simulink model "simulink_Rositani"  (R2023b)
settings: Solver=VariableStepAuto  StartTime=0.0  StopTime=10  RelTol=1e-3
values from neighbouring files (symbols this model uses):
  A_lin = [   0                       1       0       0 ... (first row only)    [main_Rositani.m]
  B_lin = [   0   0   0   1/Jm]'    [main_Rositani.m]
  Beta = sym2poly(X)    [main_Rositani.m]
  Beta_integrator = sym2poly(X_integrator)    [main_Rositani.m]
  Bl = 0    [main_Rositani.m]
  Bm = 0.015    [main_Rositani.m]
  C_lin = [   1   0   0   0]    [main_Rositani.m]
  Cfl = [1 0 0 0]    [main_Rositani.m]
  Cfl_ext = [Cfl 0]    [main_Rositani.m]
  D_lin = 0    [main_Rositani.m]
  Dfl = 0    [main_Rositani.m]
  g = 9.8    [main_Rositani.m]
  Jl = 4e-4    (= 0.0004)    [main_Rositani.m]
  Jm = Jl    (= 0.0004)    [main_Rositani.m]
  k = 0.8    [main_Rositani.m]
  Kobs = place(A_lin',C_lin',[-200,-250,-300,-350])'    [main_Rositani.m]
  Kobsfl = place(M',Cfl',[-200,-250,-300,-350])'    [main_Rositani.m]
  Kobsfl_VSCext = place(M_VSCext',Cfl_ext',[-200,-250,-300,-350,-400])'    [main_Rositani.m]
  kppext = place(Aext,Bext,[-20 -25 -30 -35 -40])    [main_Rositani.m]
  kppext_fl = place(Mext,Next,[-20 -25 -30 -35 -40])    [main_Rositani.m]
  l = 0.3    [main_Rositani.m]
  M = [0 1 0 0;0 0 1 0; 0 0 0 1; 0 0 0 0]    [main_Rositani.m]
  m = 0.3    [main_Rositani.m]
  M_VSCext = [M N;zeros(1,5)]    [main_Rositani.m]
  N = [0;0;0;1]    [main_Rositani.m]
  q = 10    [main_Rositani.m]
  r = 100    [main_Rositani.m]
  step_amp = pi/4+pi/8    (= 1.1780972451)    [main_Rositani.m]
  u_bar = m*g*l*cos(pi/4)    [main_Rositani.m]
  x0 = [x1_bar,0,x3_bar,0]'    [main_Rositani.m]
  x1_bar = pi/4    (= 0.785398163397)    [main_Rositani.m]
  x3_bar = m*g*l/k*cos(pi/4)+pi/4    [main_Rositani.m]
settings Model: Creator=gtost  LastModifiedBy=marco
settings SolverCC: ZeroCrossAlgorithm=Adaptive
settings OptimizationCC: ReuseModelBlockBuffer=off
settings DebuggingCC: MaskedZcDiagnostic=none  IgnoredZcDiagnostic=none

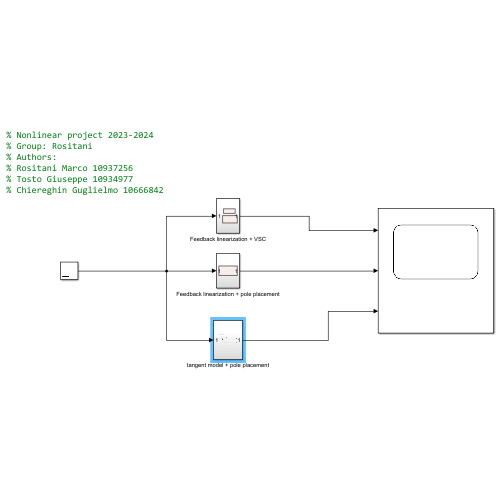
[thumbnail: Simulink's stored preview of the top-level diagram]
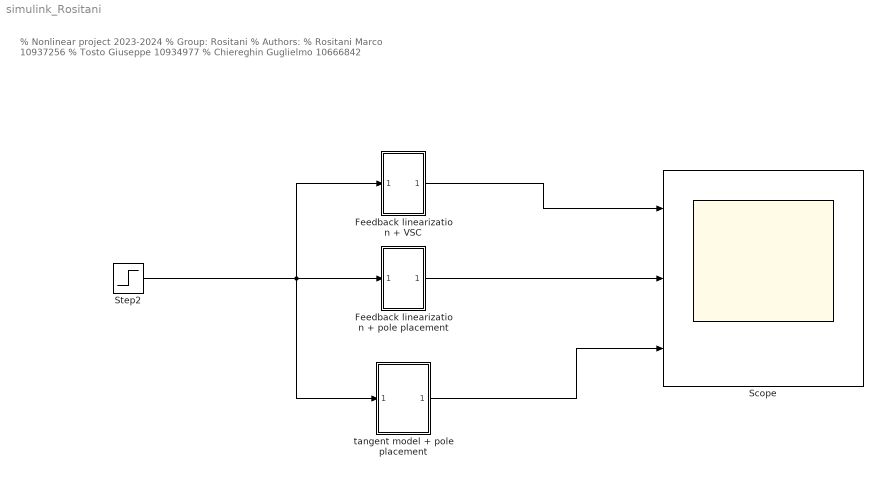
== system simulink_Rositani ==
  note: % Nonlinear project 2023-2024
      | % Group: Rositani
      | % Authors:
      | % Rositani Marco 10937256
      | % Tosto Giuseppe 10934977
      | % Chiereghin Guglielmo 10666842
  Feedback linearization + VSC : Subsystem
  Feedback linearization + pole placement : Subsystem
  Scope : Scope  NumInputPorts=3
  Step2 : Step  After=step_amp  SampleTime=0
  tangent model + pole placement : Subsystem
  wires:
  Feedback linearization + pole placement/1(Out1) -> Scope/2
  Feedback linearization + VSC/1(Out2) -> Scope/1
  tangent model + pole placement/1(Out1) -> Scope/3
  Step2/1 -> Feedback linearization + pole placement/1(Input), tangent model + pole placement/1(Input), Feedback linearization + VSC/1(Input)

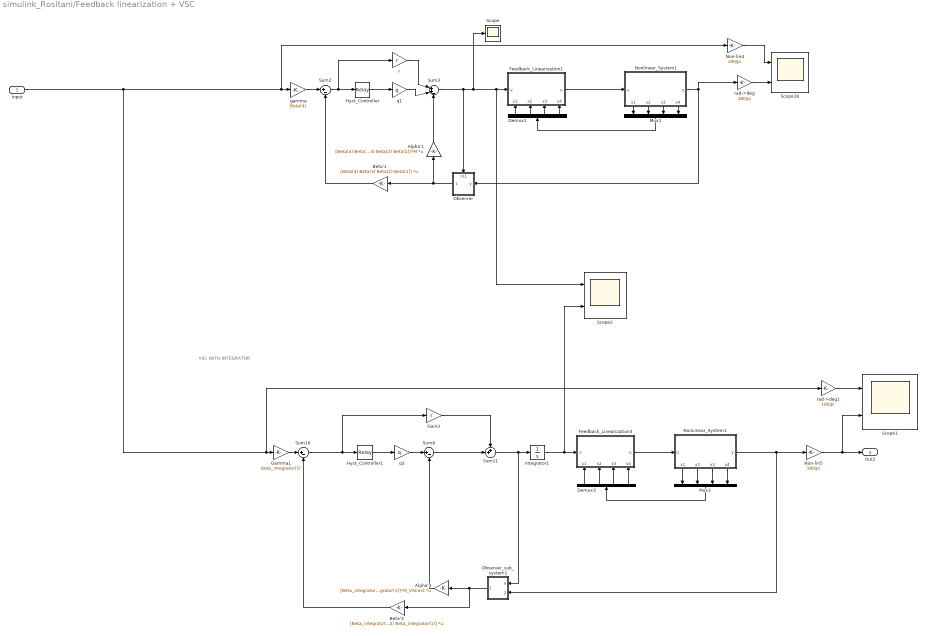
== system simulink_Rositani/Feedback linearization + VSC ==
  note: VSC WITH INTEGRATOR
  Input : Inport
  Alpha'1 : Gain  Gain=[Beta(4) Beta(3) Beta(2) Beta(1)]*M  Multiplication=Matrix(K*u)
  Alpha'3 : Gain  Gain=[Beta_integrator(5) Beta_integrator(4) Beta_integrator(3) Beta_integrator(2) Beta_integrator(1)]*M_VSCext  Multiplication=Matrix(K*u)
  Beta'1 : Gain  Gain=[Beta(4) Beta(3) Beta(2) Beta(1)]  Multiplication=Matrix(K*u)
  Beta'3 : Gain  Gain=[Beta_integrator(5) Beta_integrator(4) Beta_integrator(3) Beta_integrator(2) Beta_integrator(1)]  Multiplication=Matrix(K*u)
  Demux1 : Demux
  Demux3 : Demux
  Feedback_Linearization1 : Subsystem
      settings: PortSchema="{\"entries\":[{\"content\":{\"sides\":[{\"content\":{\"connectorIds\":[\"In1\",\"In2\",\"In3\",\"In4\"]},\"type\":\"ConnectorPlacement.EquallySpacedRectSide\",\"uuid\":\"adbcf6e9-d4ea-42de-99ff-13edcb3b1819\"},{\"content\":{\"connectorIds\":[],\"side\":\"RIGHT\"},\"type\":\"ConnectorPlacement.EquallySpacedRectSide\",\"uuid\":\"b525c529-ac30-4eee-aa98-8a0e478b5fb8\"},{\"content\":{\"connectorIds\":[\"In5\"],\"side\":\"TOP\"},\"type\":\"ConnectorPlacement.EquallySpacedRectSide\",\"uuid\":\"f99f0ac5-025d-4a5c-b3b2-d4280c578d78\"},{\"content\":{\"connectorIds\":[\"Out1\"],\"side\":\"BOTTOM\"},\"type\":\"ConnectorPlacement.EquallySpacedRectSide\",\"uuid\":\"0062a15c-7fea-4434-a819-637327a8425c\"}]},\"type\":\"ConnectorPlacement.EquallySpacedConnector\",\"uuid\":\"4fadabde-502f-417b-a41d-67ea1bbf08a5\"}],\"packageUris\":[\"http://schema.mathworks.com/mf0/Connector/R2020b\"],\"version\":\"1.0\"}"
  Feedback_Linearization3 : Subsystem
      settings: PortSchema="{\"entries\":[{\"content\":{\"sides\":[{\"content\":{\"connectorIds\":[\"In1\",\"In2\",\"In3\",\"In4\"]},\"type\":\"ConnectorPlacement.EquallySpacedRectSide\",\"uuid\":\"adbcf6e9-d4ea-42de-99ff-13edcb3b1819\"},{\"content\":{\"connectorIds\":[],\"side\":\"RIGHT\"},\"type\":\"ConnectorPlacement.EquallySpacedRectSide\",\"uuid\":\"b525c529-ac30-4eee-aa98-8a0e478b5fb8\"},{\"content\":{\"connectorIds\":[\"In5\"],\"side\":\"TOP\"},\"type\":\"ConnectorPlacement.EquallySpacedRectSide\",\"uuid\":\"f99f0ac5-025d-4a5c-b3b2-d4280c578d78\"},{\"content\":{\"connectorIds\":[\"Out1\"],\"side\":\"BOTTOM\"},\"type\":\"ConnectorPlacement.EquallySpacedRectSide\",\"uuid\":\"0062a15c-7fea-4434-a819-637327a8425c\"}]},\"type\":\"ConnectorPlacement.EquallySpacedConnector\",\"uuid\":\"4fadabde-502f-417b-a41d-67ea1bbf08a5\"}],\"packageUris\":[\"http://schema.mathworks.com/mf0/Connector/R2020b\"],\"version\":\"1.0\"}"
  Gain3 : Gain  Gain=r
  Gamma1 : Gain  Gain=Beta_integrator(5)
  Hyst_Controller : Relay  OnSwitchValue=0.2  OffSwitchValue=-0.2  OffOutputValue=-1
  Hyst_Controller1 : Relay  OnSwitchValue=0.2  OffSwitchValue=-0.2  OffOutputValue=-1
  Integrator1 : Integrator
  Mux1 : Mux
  Mux3 : Mux
  Non-lin4 : Gain  Gain=180/pi
  Non-lin5 : Gain  Gain=180/pi
  NonLInear_System1 : Subsystem
      settings: PortSchema="{\"entries\":[{\"content\":{\"sides\":[{\"content\":{\"connectorIds\":[]},\"type\":\"ConnectorPlacement.EquallySpacedRectSide\",\"uuid\":\"fc0e07bd-457d-4f73-a9de-b189f04b7406\"},{\"content\":{\"connectorIds\":[\"Out1\",\"Out2\",\"Out3\",\"Out4\"],\"side\":\"RIGHT\"},\"type\":\"ConnectorPlacement.EquallySpacedRectSide\",\"uuid\":\"a5405dd1-72e2-47e5-bf61-3afb592fd614\"},{\"content\":{\"connectorIds\":[\"In1\"],\"side\":\"TOP\"},\"type\":\"ConnectorPlacement.EquallySpacedRectSide\",\"uuid\":\"aa9f9cfa-860e-40f5-842c-a49042685ea7\"},{\"content\":{\"connectorIds\":[\"Out5\"],\"side\":\"BOTTOM\"},\"type\":\"ConnectorPlacement.EquallySpacedRectSide\",\"uuid\":\"187ae16a-996b-4444-8d39-d1043468c76c\"}]},\"type\":\"ConnectorPlacement.EquallySpacedConnector\",\"uuid\":\"6dd1d8f9-1d62-4e9a-bec2-4b959d6b58c0\"}],\"packageUris\":[\"http://schema.mathworks.com/mf0/Connector/R2020b\"],\"version\":\"1.0\"}"
  Nonlinear_System1 : Subsystem
      settings: PortSchema="{\"entries\":[{\"content\":{\"sides\":[{\"content\":{\"connectorIds\":[]},\"type\":\"ConnectorPlacement.EquallySpacedRectSide\",\"uuid\":\"fc0e07bd-457d-4f73-a9de-b189f04b7406\"},{\"content\":{\"connectorIds\":[\"Out1\",\"Out2\",\"Out3\",\"Out4\"],\"side\":\"RIGHT\"},\"type\":\"ConnectorPlacement.EquallySpacedRectSide\",\"uuid\":\"a5405dd1-72e2-47e5-bf61-3afb592fd614\"},{\"content\":{\"connectorIds\":[\"In1\"],\"side\":\"TOP\"},\"type\":\"ConnectorPlacement.EquallySpacedRectSide\",\"uuid\":\"aa9f9cfa-860e-40f5-842c-a49042685ea7\"},{\"content\":{\"connectorIds\":[\"Out5\"],\"side\":\"BOTTOM\"},\"type\":\"ConnectorPlacement.EquallySpacedRectSide\",\"uuid\":\"187ae16a-996b-4444-8d39-d1043468c76c\"}]},\"type\":\"ConnectorPlacement.EquallySpacedConnector\",\"uuid\":\"6dd1d8f9-1d62-4e9a-bec2-4b959d6b58c0\"}],\"packageUris\":[\"http://schema.mathworks.com/mf0/Connector/R2020b\"],\"version\":\"1.0\"}"
  Observer : Subsystem
      settings: PortSchema="{\"entries\":[{\"content\":{\"sides\":[{\"content\":{\"connectorIds\":[\"In1\"]},\"type\":\"ConnectorPlacement.EquallySpacedRectSide\",\"uuid\":\"2b2df3d8-1279-46b4-93b2-b5e918df1143\"},{\"content\":{\"connectorIds\":[\"Out1\"],\"side\":\"RIGHT\"},\"type\":\"ConnectorPlacement.EquallySpacedRectSide\",\"uuid\":\"29834a7d-bd18-478f-8842-72b452eb8ac1\"},{\"content\":{\"connectorIds\":[\"In2\"],\"side\":\"TOP\"},\"type\":\"ConnectorPlacement.EquallySpacedRectSide\",\"uuid\":\"8e28432d-3188-4e3a-b594-25bb706f296d\"}]},\"type\":\"ConnectorPlacement.EquallySpacedConnector\",\"uuid\":\"3baf92a3-067b-448e-904e-78e17b82779c\"}],\"packageUris\":[\"http://schema.mathworks.com/mf0/Connector/R2020b\"],\"version\":\"1.0\"}"
  Observer_sub_system1 : Subsystem
  Scope : Scope
  Scope1 : Scope  NumInputPorts=2
  Scope18 : Scope  NumInputPorts=2
  Scope2 : Scope  NumInputPorts=2
  Sum10 : Sum  Inputs=|+-
  Sum11 : Sum  Inputs=++|
  Sum2 : Sum  Inputs=|+-
  Sum3 : Sum  Inputs=|++-
  Sum8 : Sum  Inputs=|+-
  gamma : Gain  Gain=Beta(4)
  q1 : Gain  Gain=q
  q3 : Gain  Gain=q
  r : Gain  Gain=r
  rad->deg : Gain  Gain=180/pi
  rad->deg1 : Gain  Gain=180/pi
  Out2 : Outport
  wires:
  Non-lin4/1 -> Scope18/1
  Beta'1/1 -> Sum2/2
  rad->deg/1 -> Scope18/2
  Hyst_Controller/1 -> q1/1
  gamma/1 -> Sum2/1
  Nonlinear_System1/5(y) -> rad->deg/1, Observer/1(y)
  Nonlinear_System1/2(x2) -> Mux1/2
  Input/1 -> Non-lin4/1, gamma/1, rad->deg1/1, Gamma1/1
  Sum2/1 -> r/1, Hyst_Controller/1
  q1/1 -> Sum3/2
  Sum3/1 -> Observer/2(In1), Scope2/1, Feedback_Linearization1/5(v), Scope/1
  Mux1/1 -> Demux1/1
  Observer/1(Out1) -> Beta'1/1, Alpha'1/1
  Alpha'1/1 -> Sum3/3
  Nonlinear_System1/3(x3) -> Mux1/3
  Demux1/1 -> Feedback_Linearization1/1(x1)
  Nonlinear_System1/1(x1) -> Mux1/1
  r/1 -> Sum3/1
  Demux1/3 -> Feedback_Linearization1/3(x3)
  Demux1/2 -> Feedback_Linearization1/2(x2)
  Demux1/4 -> Feedback_Linearization1/4(x4)
  Nonlinear_System1/4(x4) -> Mux1/4
  Feedback_Linearization1/1(u) -> Nonlinear_System1/1(u)
  Alpha'3/1 -> Sum8/2
  Feedback_Linearization3/1(u) -> NonLInear_System1/1(u)
  Sum11/1 -> Integrator1/1, Observer_sub_system1/1(u)
  q3/1 -> Sum8/1
  Hyst_Controller1/1 -> q3/1
  Gamma1/1 -> Sum10/1
  Non-lin5/1 -> Scope1/2, Out2/1
  NonLInear_System1/3(x3) -> Mux3/3
  Gain3/1 -> Sum11/1
  NonLInear_System1/5(y) -> Observer_sub_system1/2(Input), Non-lin5/1
  Observer_sub_system1/1(Out1) -> Alpha'3/1, Beta'3/1
  Sum10/1 -> Hyst_Controller1/1, Gain3/1
  Demux3/2 -> Feedback_Linearization3/2(x2)
  NonLInear_System1/2(x2) -> Mux3/2
  NonLInear_System1/4(x4) -> Mux3/4
  Demux3/3 -> Feedback_Linearization3/3(x3)
  Mux3/1 -> Demux3/1
  Beta'3/1 -> Sum10/2
  Demux3/1 -> Feedback_Linearization3/1(x1)
  Sum8/1 -> Sum11/2
  NonLInear_System1/1(x1) -> Mux3/1
  Demux3/4 -> Feedback_Linearization3/4(x4)
  rad->deg1/1 -> Scope1/1
  Integrator1/1 -> Scope2/2, Feedback_Linearization3/5(v)

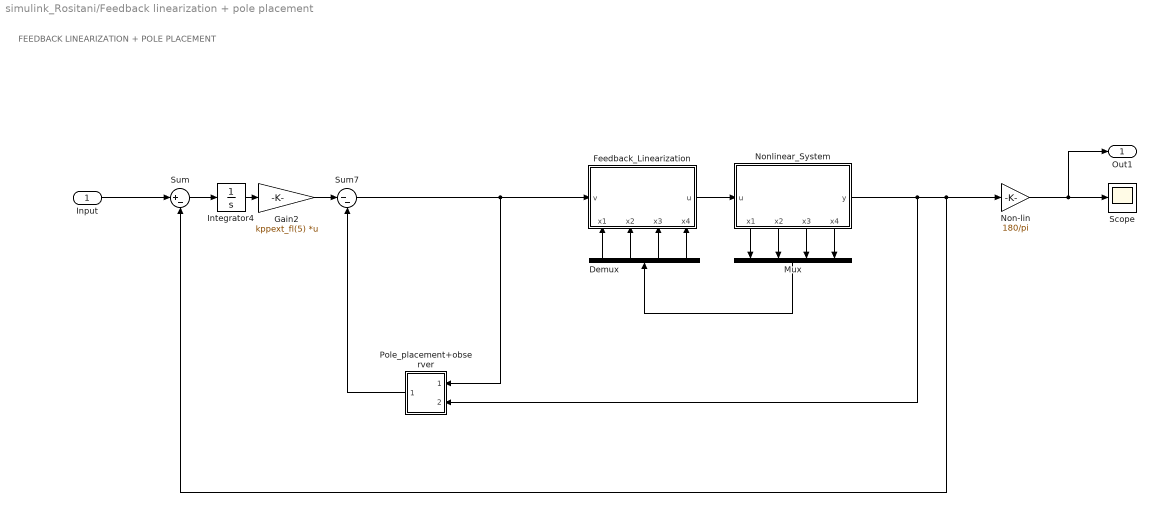
== system simulink_Rositani/Feedback linearization + pole placement ==
  note: FEEDBACK LINEARIZATION + POLE PLACEMENT
  Input : Inport
  Demux : Demux
  Feedback_Linearization : Subsystem
      settings: PortSchema="{\"entries\":[{\"content\":{\"sides\":[{\"content\":{\"connectorIds\":[\"In1\",\"In2\",\"In3\",\"In4\"]},\"type\":\"ConnectorPlacement.EquallySpacedRectSide\",\"uuid\":\"adbcf6e9-d4ea-42de-99ff-13edcb3b1819\"},{\"content\":{\"side\":\"RIGHT\"},\"type\":\"ConnectorPlacement.EquallySpacedRectSide\",\"uuid\":\"b525c529-ac30-4eee-aa98-8a0e478b5fb8\"},{\"content\":{\"connectorIds\":[\"In5\"],\"side\":\"TOP\"},\"type\":\"ConnectorPlacement.EquallySpacedRectSide\",\"uuid\":\"f99f0ac5-025d-4a5c-b3b2-d4280c578d78\"},{\"content\":{\"connectorIds\":[\"Out1\"],\"side\":\"BOTTOM\"},\"type\":\"ConnectorPlacement.EquallySpacedRectSide\",\"uuid\":\"0062a15c-7fea-4434-a819-637327a8425c\"}]},\"type\":\"ConnectorPlacement.EquallySpacedConnector\",\"uuid\":\"4fadabde-502f-417b-a41d-67ea1bbf08a5\"}],\"packageUris\":[\"http://schema.mathworks.com/mf0/Connector/R2020b\"],\"version\":\"1.0\"}"
  Gain2 : Gain  Gain=kppext_fl(5)  Multiplication=Matrix(K*u) (u vector)
  Integrator4 : Integrator
  Mux : Mux
  Non-lin : Gain  Gain=180/pi
  Nonlinear_System : Subsystem
      settings: PortSchema="{\"entries\":[{\"content\":{\"sides\":[{\"content\":{\"connectorIds\":[]},\"type\":\"ConnectorPlacement.EquallySpacedRectSide\",\"uuid\":\"fc0e07bd-457d-4f73-a9de-b189f04b7406\"},{\"content\":{\"connectorIds\":[\"Out1\",\"Out2\",\"Out3\",\"Out4\"],\"side\":\"RIGHT\"},\"type\":\"ConnectorPlacement.EquallySpacedRectSide\",\"uuid\":\"a5405dd1-72e2-47e5-bf61-3afb592fd614\"},{\"content\":{\"connectorIds\":[\"In1\"],\"side\":\"TOP\"},\"type\":\"ConnectorPlacement.EquallySpacedRectSide\",\"uuid\":\"aa9f9cfa-860e-40f5-842c-a49042685ea7\"},{\"content\":{\"connectorIds\":[\"Out5\"],\"side\":\"BOTTOM\"},\"type\":\"ConnectorPlacement.EquallySpacedRectSide\",\"uuid\":\"187ae16a-996b-4444-8d39-d1043468c76c\"}]},\"type\":\"ConnectorPlacement.EquallySpacedConnector\",\"uuid\":\"6dd1d8f9-1d62-4e9a-bec2-4b959d6b58c0\"}],\"packageUris\":[\"http://schema.mathworks.com/mf0/Connector/R2020b\"],\"version\":\"1.0\"}"
  Pole_placement+observer : Subsystem
  Scope : Scope
  Sum : Sum  Inputs=|+-
  Sum7 : Sum  Inputs=|--
  Out1 : Outport
  wires:
  Nonlinear_System/2(x2) -> Mux/2
  Demux/1 -> Feedback_Linearization/1(x1)
  Demux/4 -> Feedback_Linearization/4(x4)
  Pole_placement+observer/1(Out1) -> Sum7/2
  Nonlinear_System/1(x1) -> Mux/1
  Gain2/1 -> Sum7/1
  Sum7/1 -> Pole_placement+observer/1(In1), Feedback_Linearization/5(v)
  Nonlinear_System/4(x4) -> Mux/4
  Nonlinear_System/3(x3) -> Mux/3
  Demux/3 -> Feedback_Linearization/3(x3)
  Demux/2 -> Feedback_Linearization/2(x2)
  Sum/1 -> Integrator4/1
  Nonlinear_System/5(y) -> Pole_placement+observer/2(Input), Sum/2, Non-lin/1
  Integrator4/1 -> Gain2/1
  Feedback_Linearization/1(u) -> Nonlinear_System/1(u)
  Non-lin/1 -> Scope/1, Out1/1
  Input/1 -> Sum/1
  Mux/1 -> Demux/1

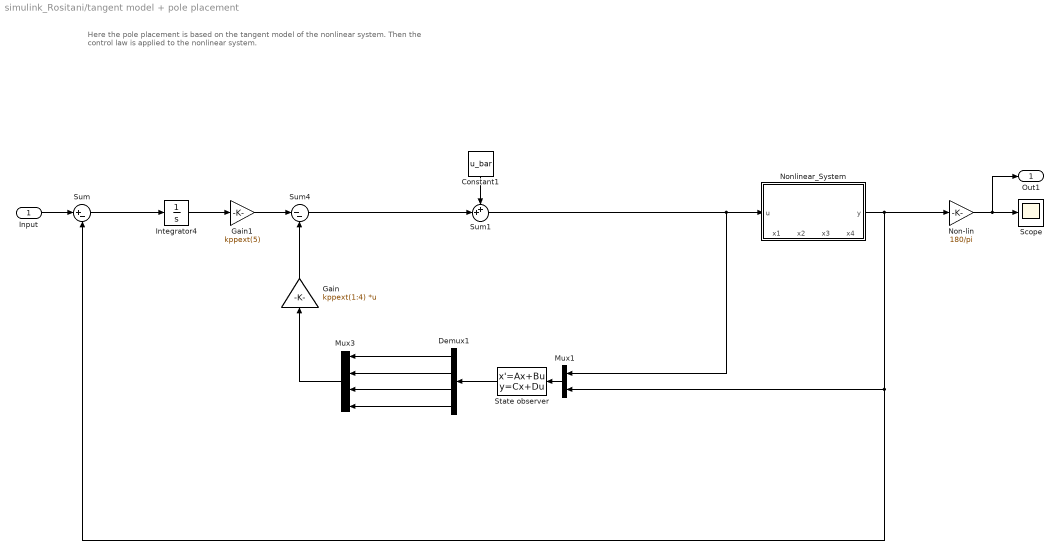
== system simulink_Rositani/tangent model + pole placement ==
  note: Here the pole placement is based on the tangent model of the nonlinear system. Then the control law is applied to the nonlinear system.
  Input : Inport
  Constant1 : Constant  Value=u_bar
  Demux1 : Demux
  Gain : Gain  Gain=kppext(1:4)  Multiplication=Matrix(K*u) (u vector)
  Gain1 : Gain  Gain=kppext(5)
  Integrator4 : Integrator
  Mux1 : Mux  Inputs=2
  Mux3 : Mux
  Non-lin : Gain  Gain=180/pi
  Nonlinear_System : Subsystem
      settings: PortSchema="{\"entries\":[{\"content\":{\"sides\":[{\"content\":{\"connectorIds\":[]},\"type\":\"ConnectorPlacement.EquallySpacedRectSide\",\"uuid\":\"fc0e07bd-457d-4f73-a9de-b189f04b7406\"},{\"content\":{\"connectorIds\":[\"Out1\",\"Out2\",\"Out3\",\"Out4\"],\"side\":\"RIGHT\"},\"type\":\"ConnectorPlacement.EquallySpacedRectSide\",\"uuid\":\"a5405dd1-72e2-47e5-bf61-3afb592fd614\"},{\"content\":{\"connectorIds\":[\"In1\"],\"side\":\"TOP\"},\"type\":\"ConnectorPlacement.EquallySpacedRectSide\",\"uuid\":\"aa9f9cfa-860e-40f5-842c-a49042685ea7\"},{\"content\":{\"connectorIds\":[\"Out5\"],\"side\":\"BOTTOM\"},\"type\":\"ConnectorPlacement.EquallySpacedRectSide\",\"uuid\":\"187ae16a-996b-4444-8d39-d1043468c76c\"}]},\"type\":\"ConnectorPlacement.EquallySpacedConnector\",\"uuid\":\"6dd1d8f9-1d62-4e9a-bec2-4b959d6b58c0\"}],\"packageUris\":[\"http://schema.mathworks.com/mf0/Connector/R2020b\"],\"version\":\"1.0\"}"
  Scope : Scope
  State observer : StateSpace  A=A_lin-Kobs*C_lin  B=[B_lin-Kobs*D_lin Kobs]  C=eye(4)  D=[0 0;0 0;0 0;0 0]  InitialCondition=0  ParameterTunability=Unconstrained
  Sum : Sum  Inputs=|+-
  Sum1 : Sum  Inputs=++|
  Sum4 : Sum  Inputs=|--
  Out1 : Outport
  wires:
  Sum4/1 -> Sum1/2
  Constant1/1 -> Sum1/1
  Sum1/1 -> Mux1/1, Nonlinear_System/1(u)
  State observer/1 -> Demux1/1
  Demux1/2 -> Mux3/2
  Demux1/4 -> Mux3/4
  Gain/1 -> Sum4/2
  Nonlinear_System/5(y) -> Non-lin/1, Sum/2, Mux1/2
  Sum/1 -> Integrator4/1
  Integrator4/1 -> Gain1/1
  Gain1/1 -> Sum4/1
  Mux1/1 -> State observer/1
  Demux1/1 -> Mux3/1
  Demux1/3 -> Mux3/3
  Non-lin/1 -> Out1/1, Scope/1
  Mux3/1 -> Gain/1
  Input/1 -> Sum/1

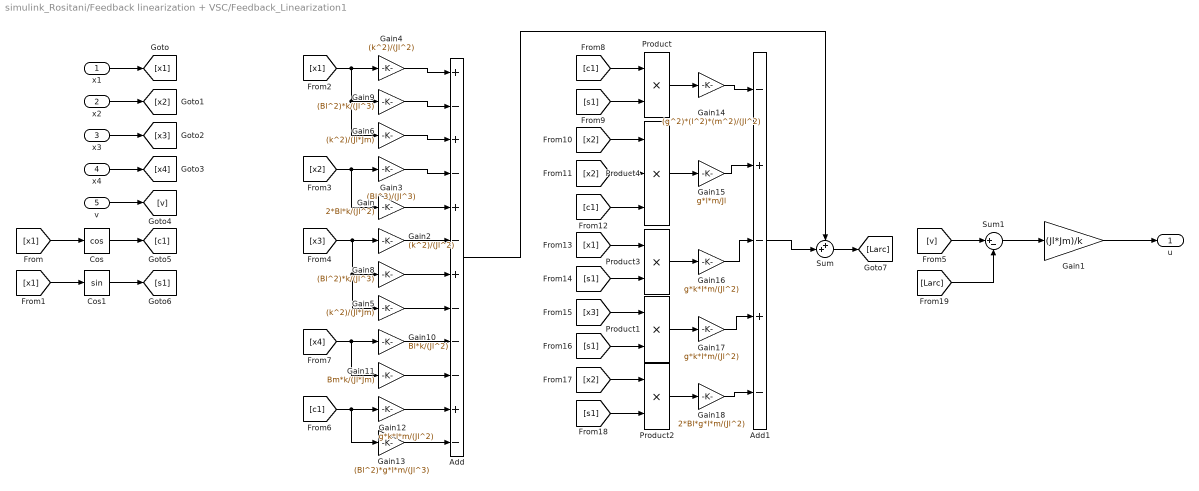
== system simulink_Rositani/Feedback linearization + VSC/Feedback_Linearization1 ==
  x1 : Inport
  x2 : Inport  Port=2
  x3 : Inport  Port=3
  x4 : Inport  Port=4
  v : Inport  Port=5
  Add : Sum  Inputs=+-+-+-+---+-
  Add1 : Sum  Inputs=-+-+-
  Cos : Trigonometry  Operator=cos
  Cos1 : Trigonometry
  Gain : Gain  Gain=2*Bl*k/(Jl^2)
  Gain1 : Gain  Gain=(Jl*Jm)/k
  Gain10 : Gain  Gain=Bl*k/(Jl^2)
  Gain11 : Gain  Gain=Bm*k/(Jl*Jm)
  Gain12 : Gain  Gain=g*k*l*m/(Jl^2)
  Gain13 : Gain  Gain=(Bl^2)*g*l*m/(Jl^3)
  Gain14 : Gain  Gain=(g^2)*(l^2)*(m^2)/(Jl^2)
  Gain15 : Gain  Gain=g*l*m/Jl
  Gain16 : Gain  Gain=g*k*l*m/(Jl^2)
  Gain17 : Gain  Gain=g*k*l*m/(Jl^2)
  Gain18 : Gain  Gain=2*Bl*g*l*m/(Jl^2)
  Gain2 : Gain  Gain=(k^2)/(Jl^2)
  Gain3 : Gain  Gain=(Bl^3)/(Jl^3)
  Gain4 : Gain  Gain=(k^2)/(Jl^2)
  Gain5 : Gain  Gain=(k^2)/(Jl*Jm)
  Gain6 : Gain  Gain=(k^2)/(Jl*Jm)
  Gain8 : Gain  Gain=(Bl^2)*k/(Jl^3)
  Gain9 : Gain  Gain=(Bl^2)*k/(Jl^3)
  Product{,1..3} (4 alike) : Product
  Product4 : Product  Inputs=3
  Sum : Sum  Inputs=++|
  Sum1 : Sum  Inputs=|+-
  u : Outport
  wires:
  x1/1 -> [x1]
  x2/1 -> [x2]
  x3/1 -> [x3]
  x4/1 -> [x4]
  v/1 -> [v]
  [x1] -> Cos/1
  Cos/1 -> [c1]
  Cos1/1 -> [s1]
  [x1] -> Cos1/1
  [x2] -> Gain/1, Gain3/1
  [x1] -> Gain6/1, Gain9/1, Gain4/1
  [x3] -> Gain5/1, Gain8/1, Gain2/1
  [x4] -> Gain11/1, Gain10/1
  [c1] -> Gain13/1, Gain12/1
  [c1] -> Product/1
  [s1] -> Product/2
  Product/1 -> Gain14/1
  [x2] -> Product4/1
  [x2] -> Product4/2
  [c1] -> Product4/3
  Product4/1 -> Gain15/1
  [x1] -> Product3/1
  [s1] -> Product3/2
  [x3] -> Product1/1
  [s1] -> Product1/2
  [x2] -> Product2/1
  [s1] -> Product2/2
  Product3/1 -> Gain16/1
  Product1/1 -> Gain17/1
  Product2/1 -> Gain18/1
  Gain4/1 -> Add/1
  Gain9/1 -> Add/2
  Gain6/1 -> Add/3
  Gain3/1 -> Add/4
  Gain/1 -> Add/5
  Gain2/1 -> Add/6
  Gain8/1 -> Add/7
  Gain5/1 -> Add/8
  Gain10/1 -> Add/9
  Gain11/1 -> Add/10
  Gain12/1 -> Add/11
  Gain13/1 -> Add/12
  Gain14/1 -> Add1/1
  Gain15/1 -> Add1/2
  Gain16/1 -> Add1/3
  Gain17/1 -> Add1/4
  Gain18/1 -> Add1/5
  Add1/1 -> Sum/2
  Add/1 -> Sum/1
  Sum/1 -> [Larc]
  [v] -> Sum1/1
  [Larc] -> Sum1/2
  Sum1/1 -> Gain1/1
  Gain1/1 -> u/1

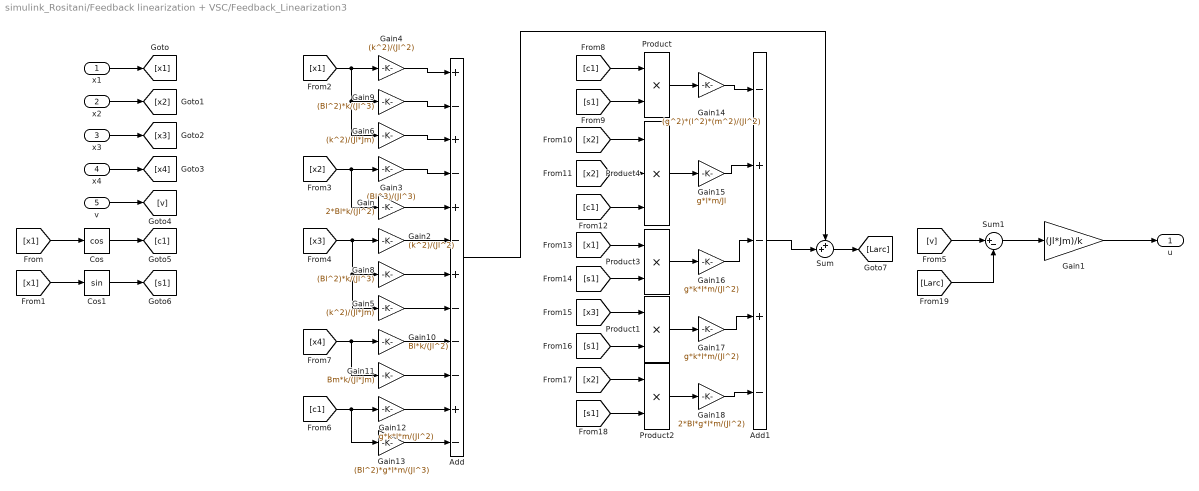
== system simulink_Rositani/Feedback linearization + VSC/Feedback_Linearization3 ==
  x1 : Inport
  x2 : Inport  Port=2
  x3 : Inport  Port=3
  x4 : Inport  Port=4
  v : Inport  Port=5
  Add : Sum  Inputs=+-+-+-+---+-
  Add1 : Sum  Inputs=-+-+-
  Cos : Trigonometry  Operator=cos
  Cos1 : Trigonometry
  Gain : Gain  Gain=2*Bl*k/(Jl^2)
  Gain1 : Gain  Gain=(Jl*Jm)/k
  Gain10 : Gain  Gain=Bl*k/(Jl^2)
  Gain11 : Gain  Gain=Bm*k/(Jl*Jm)
  Gain12 : Gain  Gain=g*k*l*m/(Jl^2)
  Gain13 : Gain  Gain=(Bl^2)*g*l*m/(Jl^3)
  Gain14 : Gain  Gain=(g^2)*(l^2)*(m^2)/(Jl^2)
  Gain15 : Gain  Gain=g*l*m/Jl
  Gain16 : Gain  Gain=g*k*l*m/(Jl^2)
  Gain17 : Gain  Gain=g*k*l*m/(Jl^2)
  Gain18 : Gain  Gain=2*Bl*g*l*m/(Jl^2)
  Gain2 : Gain  Gain=(k^2)/(Jl^2)
  Gain3 : Gain  Gain=(Bl^3)/(Jl^3)
  Gain4 : Gain  Gain=(k^2)/(Jl^2)
  Gain5 : Gain  Gain=(k^2)/(Jl*Jm)
  Gain6 : Gain  Gain=(k^2)/(Jl*Jm)
  Gain8 : Gain  Gain=(Bl^2)*k/(Jl^3)
  Gain9 : Gain  Gain=(Bl^2)*k/(Jl^3)
  Product{,1..3} (4 alike) : Product
  Product4 : Product  Inputs=3
  Sum : Sum  Inputs=++|
  Sum1 : Sum  Inputs=|+-
  u : Outport
  wires:
  x1/1 -> [x1]
  x2/1 -> [x2]
  x3/1 -> [x3]
  x4/1 -> [x4]
  v/1 -> [v]
  [x1] -> Cos/1
  Cos/1 -> [c1]
  Cos1/1 -> [s1]
  [x1] -> Cos1/1
  [x2] -> Gain/1, Gain3/1
  [x1] -> Gain6/1, Gain9/1, Gain4/1
  [x3] -> Gain5/1, Gain8/1, Gain2/1
  [x4] -> Gain11/1, Gain10/1
  [c1] -> Gain13/1, Gain12/1
  [c1] -> Product/1
  [s1] -> Product/2
  Product/1 -> Gain14/1
  [x2] -> Product4/1
  [x2] -> Product4/2
  [c1] -> Product4/3
  Product4/1 -> Gain15/1
  [x1] -> Product3/1
  [s1] -> Product3/2
  [x3] -> Product1/1
  [s1] -> Product1/2
  [x2] -> Product2/1
  [s1] -> Product2/2
  Product3/1 -> Gain16/1
  Product1/1 -> Gain17/1
  Product2/1 -> Gain18/1
  Gain4/1 -> Add/1
  Gain9/1 -> Add/2
  Gain6/1 -> Add/3
  Gain3/1 -> Add/4
  Gain/1 -> Add/5
  Gain2/1 -> Add/6
  Gain8/1 -> Add/7
  Gain5/1 -> Add/8
  Gain10/1 -> Add/9
  Gain11/1 -> Add/10
  Gain12/1 -> Add/11
  Gain13/1 -> Add/12
  Gain14/1 -> Add1/1
  Gain15/1 -> Add1/2
  Gain16/1 -> Add1/3
  Gain17/1 -> Add1/4
  Gain18/1 -> Add1/5
  Add1/1 -> Sum/2
  Add/1 -> Sum/1
  Sum/1 -> [Larc]
  [v] -> Sum1/1
  [Larc] -> Sum1/2
  Sum1/1 -> Gain1/1
  Gain1/1 -> u/1

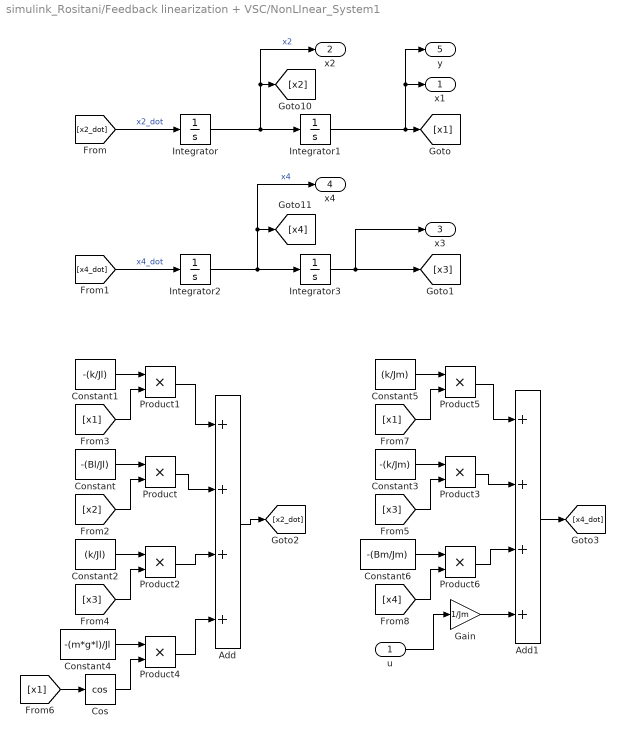
== system simulink_Rositani/Feedback linearization + VSC/NonLInear_System1 ==
  u : Inport
  Add : Sum  Inputs=++++
  Add1 : Sum  Inputs=++++
  Constant : Constant  Value=-(Bl/Jl)
  Constant1 : Constant  Value=-(k/Jl)
  Constant2 : Constant  Value=(k/Jl)
  Constant3 : Constant  Value=-(k/Jm)
  Constant4 : Constant  Value=-(m*g*l)/Jl
  Constant5 : Constant  Value=(k/Jm)
  Constant6 : Constant  Value=-(Bm/Jm)
  Cos : Trigonometry  Operator=cos
  Gain : Gain  Gain=1/Jm
  Integrator : Integrator  InitialCondition=x0(2)
  Integrator1 : Integrator  InitialCondition=x0(1)
  Integrator2 : Integrator  InitialCondition=x0(4)
  Integrator3 : Integrator  InitialCondition=x0(3)
  Product{,1..6} (7 alike) : Product
  x1 : Outport
  x2 : Outport  Port=2
  x3 : Outport  Port=3
  x4 : Outport  Port=4
  y : Outport  Port=5
  wires:
  [x2] -> Product/2
  [x2_dot] -> Integrator/1  "x2_dot"
  [x1] -> Product1/2
  Constant2/1 -> Product2/1
  [x1] -> Product5/2
  Product1/1 -> Add/1
  [x4] -> Product6/2
  Product3/1 -> Add1/2
  Integrator3/1 -> x3/1, [x3]
  [x4_dot] -> Integrator2/1  "x4_dot"
  [x3] -> Product2/2
  Constant6/1 -> Product6/1
  Cos/1 -> Product4/2
  Integrator1/1 -> y/1, x1/1, [x1]
  Integrator2/1 -> x4/1, [x4], Integrator3/1  "x4"
  Constant/1 -> Product/1
  Integrator/1 -> x2/1, [x2], Integrator1/1  "x2"
  [x1] -> Cos/1
  Product5/1 -> Add1/1
  Constant3/1 -> Product3/1
  Constant5/1 -> Product5/1
  Product/1 -> Add/2
  Product6/1 -> Add1/3
  Product2/1 -> Add/3
  Add/1 -> [x2_dot]
  [x3] -> Product3/2
  Product4/1 -> Add/4
  Add1/1 -> [x4_dot]
  Constant4/1 -> Product4/1
  Constant1/1 -> Product1/1
  Gain/1 -> Add1/4
  u/1 -> Gain/1

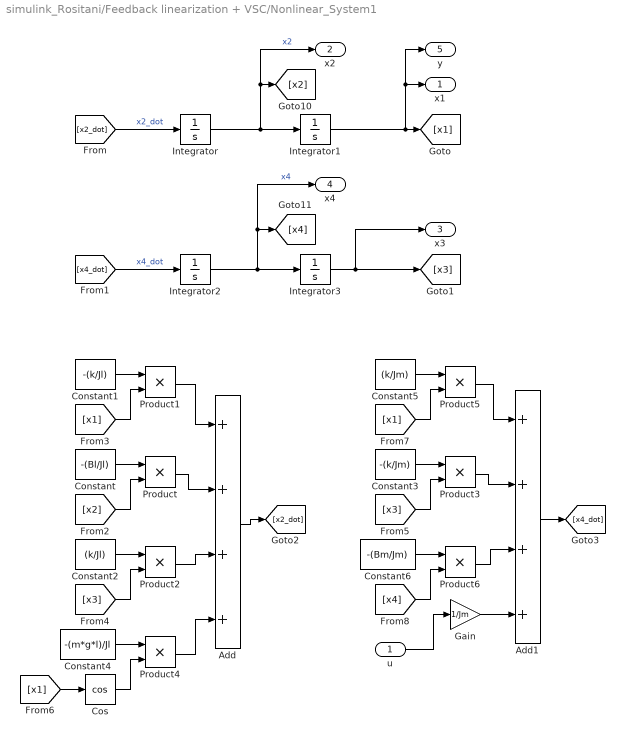
== system simulink_Rositani/Feedback linearization + VSC/Nonlinear_System1 ==
  u : Inport
  Add : Sum  Inputs=++++
  Add1 : Sum  Inputs=++++
  Constant : Constant  Value=-(Bl/Jl)
  Constant1 : Constant  Value=-(k/Jl)
  Constant2 : Constant  Value=(k/Jl)
  Constant3 : Constant  Value=-(k/Jm)
  Constant4 : Constant  Value=-(m*g*l)/Jl
  Constant5 : Constant  Value=(k/Jm)
  Constant6 : Constant  Value=-(Bm/Jm)
  Cos : Trigonometry  Operator=cos
  Gain : Gain  Gain=1/Jm
  Integrator : Integrator
  Integrator1 : Integrator  InitialCondition=x1_bar
  Integrator2 : Integrator
  Integrator3 : Integrator  InitialCondition=x3_bar
  Product{,1..6} (7 alike) : Product
  x1 : Outport
  x2 : Outport  Port=2
  x3 : Outport  Port=3
  x4 : Outport  Port=4
  y : Outport  Port=5
  wires:
  [x2] -> Product/2
  [x2_dot] -> Integrator/1  "x2_dot"
  [x1] -> Product1/2
  Constant2/1 -> Product2/1
  [x1] -> Product5/2
  Product1/1 -> Add/1
  [x4] -> Product6/2
  Product3/1 -> Add1/2
  Integrator3/1 -> x3/1, [x3]
  [x4_dot] -> Integrator2/1  "x4_dot"
  [x3] -> Product2/2
  Constant6/1 -> Product6/1
  Cos/1 -> Product4/2
  Integrator1/1 -> y/1, x1/1, [x1]
  Integrator2/1 -> x4/1, [x4], Integrator3/1  "x4"
  Constant/1 -> Product/1
  Integrator/1 -> x2/1, [x2], Integrator1/1  "x2"
  [x1] -> Cos/1
  Product5/1 -> Add1/1
  Constant3/1 -> Product3/1
  Constant5/1 -> Product5/1
  Product/1 -> Add/2
  Product6/1 -> Add1/3
  Product2/1 -> Add/3
  Add/1 -> [x2_dot]
  [x3] -> Product3/2
  Product4/1 -> Add/4
  Add1/1 -> [x4_dot]
  Constant4/1 -> Product4/1
  Constant1/1 -> Product1/1
  Gain/1 -> Add1/4
  u/1 -> Gain/1

== system simulink_Rositani/Feedback linearization + VSC/Observer ==
  y : Inport
  In1 : Inport  Port=2
  Demux2 : Demux
  Mux2 : Mux
  Mux3 : Mux  Inputs=2
  State observer2 : StateSpace  A=M-Kobsfl*Cfl  B=[N-Kobsfl*Dfl Kobsfl]  C=eye(4)  D=[0 0;0 0;0 0;0 0]  InitialCondition=[x1_bar 0 x3_bar 0]
  Out1 : Outport
  wires:
  Demux2/1 -> Mux2/1
  State observer2/1 -> Demux2/1
  Demux2/2 -> Mux2/2
  Mux3/1 -> State observer2/1
  Demux2/3 -> Mux2/3
  Demux2/4 -> Mux2/4
  In1/1 -> Mux3/1
  y/1 -> Mux3/2
  Mux2/1 -> Out1/1

== system simulink_Rositani/Feedback linearization + VSC/Observer_sub_system1 ==
  u : Inport
  Input : Inport  Port=2
  Demux1 : Demux  Outputs=5
  Mux1 : Mux  Inputs=5
  Mux2 : Mux  Inputs=2
  State observer2 : StateSpace  A=M_VSCext-Kobsfl_VSCext*Cfl_ext  B="[[0 0 0 0 1]'-Kobsfl_VSCext*Dfl  Kobsfl_VSCext]"  C=eye(5)  D=[0 0;0 0;0 0;0 0;0 0]  InitialCondition=[pi/4 0 x3_bar 0 0]  ParameterTunability=Unconstrained
  Out1 : Outport
  wires:
  Input/1 -> Mux2/2
  Demux1/3 -> Mux1/3
  State observer2/1 -> Demux1/1
  Demux1/1 -> Mux1/1
  Demux1/2 -> Mux1/2
  u/1 -> Mux2/1
  Mux2/1 -> State observer2/1
  Mux1/1 -> Out1/1
  Demux1/5 -> Mux1/5
  Demux1/4 -> Mux1/4

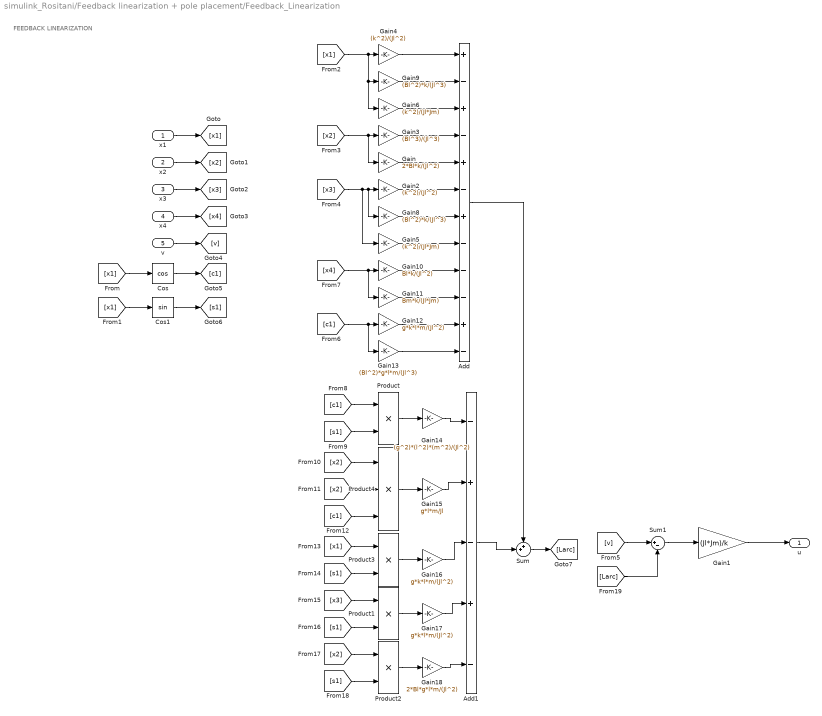
== system simulink_Rositani/Feedback linearization + pole placement/Feedback_Linearization ==
  note: FEEDBACK LINEARIZATION
  x1 : Inport
  x2 : Inport  Port=2
  x3 : Inport  Port=3
  x4 : Inport  Port=4
  v : Inport  Port=5
  Add : Sum  Inputs=+-+-+-+---+-
  Add1 : Sum  Inputs=-+-+-
  Cos : Trigonometry  Operator=cos
  Cos1 : Trigonometry
  Gain : Gain  Gain=2*Bl*k/(Jl^2)
  Gain1 : Gain  Gain=(Jl*Jm)/k
  Gain10 : Gain  Gain=Bl*k/(Jl^2)
  Gain11 : Gain  Gain=Bm*k/(Jl*Jm)
  Gain12 : Gain  Gain=g*k*l*m/(Jl^2)
  Gain13 : Gain  Gain=(Bl^2)*g*l*m/(Jl^3)
  Gain14 : Gain  Gain=(g^2)*(l^2)*(m^2)/(Jl^2)
  Gain15 : Gain  Gain=g*l*m/Jl
  Gain16 : Gain  Gain=g*k*l*m/(Jl^2)
  Gain17 : Gain  Gain=g*k*l*m/(Jl^2)
  Gain18 : Gain  Gain=2*Bl*g*l*m/(Jl^2)
  Gain2 : Gain  Gain=(k^2)/(Jl^2)
  Gain3 : Gain  Gain=(Bl^3)/(Jl^3)
  Gain4 : Gain  Gain=(k^2)/(Jl^2)
  Gain5 : Gain  Gain=(k^2)/(Jl*Jm)
  Gain6 : Gain  Gain=(k^2)/(Jl*Jm)
  Gain8 : Gain  Gain=(Bl^2)*k/(Jl^3)
  Gain9 : Gain  Gain=(Bl^2)*k/(Jl^3)
  Product{,1..3} (4 alike) : Product
  Product4 : Product  Inputs=3
  Sum : Sum  Inputs=++|
  Sum1 : Sum  Inputs=|+-
  u : Outport
  wires:
  x1/1 -> [x1]
  x2/1 -> [x2]
  x3/1 -> [x3]
  x4/1 -> [x4]
  v/1 -> [v]
  [x1] -> Cos/1
  Cos/1 -> [c1]
  Cos1/1 -> [s1]
  [x1] -> Cos1/1
  [x2] -> Gain/1, Gain3/1
  [x1] -> Gain6/1, Gain9/1, Gain4/1
  [x3] -> Gain8/1, Gain2/1, Gain5/1
  [x4] -> Gain11/1, Gain10/1
  [c1] -> Gain13/1, Gain12/1
  [c1] -> Product/1
  [s1] -> Product/2
  Product/1 -> Gain14/1
  [x2] -> Product4/1
  [x2] -> Product4/2
  [c1] -> Product4/3
  Product4/1 -> Gain15/1
  [x1] -> Product3/1
  [s1] -> Product3/2
  [x3] -> Product1/1
  [s1] -> Product1/2
  [x2] -> Product2/1
  [s1] -> Product2/2
  Product3/1 -> Gain16/1
  Product1/1 -> Gain17/1
  Product2/1 -> Gain18/1
  Gain4/1 -> Add/1
  Gain9/1 -> Add/2
  Gain6/1 -> Add/3
  Gain3/1 -> Add/4
  Gain/1 -> Add/5
  Gain2/1 -> Add/6
  Gain8/1 -> Add/7
  Gain5/1 -> Add/8
  Gain10/1 -> Add/9
  Gain11/1 -> Add/10
  Gain12/1 -> Add/11
  Gain13/1 -> Add/12
  Gain14/1 -> Add1/1
  Gain15/1 -> Add1/2
  Gain16/1 -> Add1/3
  Gain17/1 -> Add1/4
  Gain18/1 -> Add1/5
  Add1/1 -> Sum/2
  Add/1 -> Sum/1
  Sum/1 -> [Larc]
  [v] -> Sum1/1
  [Larc] -> Sum1/2
  Sum1/1 -> Gain1/1
  Gain1/1 -> u/1

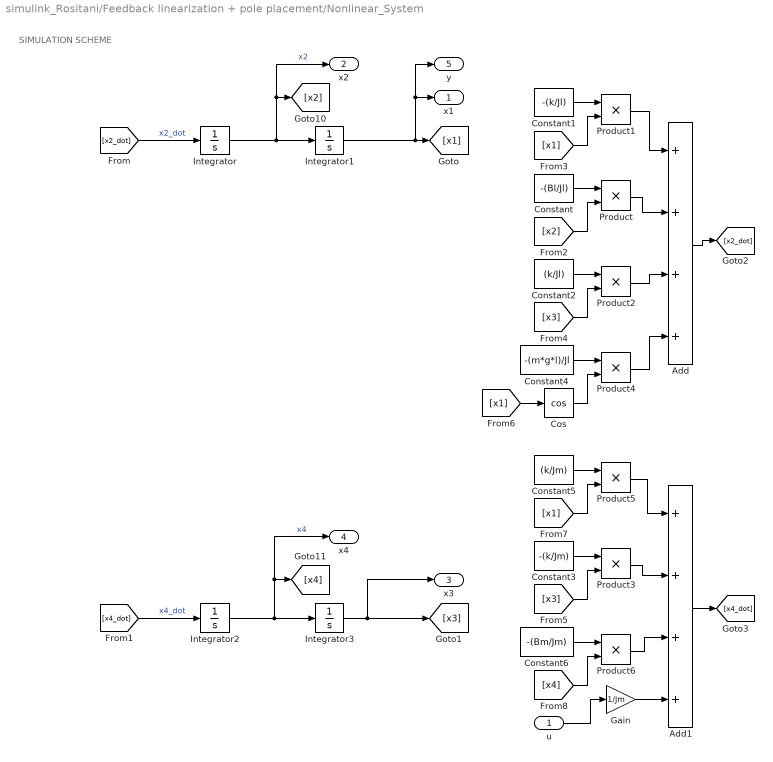
== system simulink_Rositani/Feedback linearization + pole placement/Nonlinear_System ==
  note: SIMULATION SCHEME
  u : Inport
  Add : Sum  Inputs=++++
  Add1 : Sum  Inputs=++++
  Constant : Constant  Value=-(Bl/Jl)
  Constant1 : Constant  Value=-(k/Jl)
  Constant2 : Constant  Value=(k/Jl)
  Constant3 : Constant  Value=-(k/Jm)
  Constant4 : Constant  Value=-(m*g*l)/Jl
  Constant5 : Constant  Value=(k/Jm)
  Constant6 : Constant  Value=-(Bm/Jm)
  Cos : Trigonometry  Operator=cos
  Gain : Gain  Gain=1/Jm
  Integrator : Integrator  InitialCondition=x0(2)
  Integrator1 : Integrator  InitialCondition=x0(1)
  Integrator2 : Integrator  InitialCondition=x0(4)
  Integrator3 : Integrator  InitialCondition=x0(3)
  Product{,1..6} (7 alike) : Product
  x1 : Outport
  x2 : Outport  Port=2
  x3 : Outport  Port=3
  x4 : Outport  Port=4
  y : Outport  Port=5
  wires:
  [x2] -> Product/2
  [x2_dot] -> Integrator/1  "x2_dot"
  [x1] -> Product1/2
  Constant2/1 -> Product2/1
  [x1] -> Product5/2
  Product1/1 -> Add/1
  [x4] -> Product6/2
  Product3/1 -> Add1/2
  Integrator3/1 -> x3/1, [x3]
  [x4_dot] -> Integrator2/1  "x4_dot"
  [x3] -> Product2/2
  Constant6/1 -> Product6/1
  Cos/1 -> Product4/2
  Integrator1/1 -> y/1, x1/1, [x1]
  Integrator2/1 -> x4/1, [x4], Integrator3/1  "x4"
  Constant/1 -> Product/1
  Integrator/1 -> x2/1, [x2], Integrator1/1  "x2"
  [x1] -> Cos/1
  Product5/1 -> Add1/1
  Constant3/1 -> Product3/1
  Constant5/1 -> Product5/1
  Product/1 -> Add/2
  Product6/1 -> Add1/3
  Product2/1 -> Add/3
  Add/1 -> [x2_dot]
  [x3] -> Product3/2
  Product4/1 -> Add/4
  Add1/1 -> [x4_dot]
  Constant4/1 -> Product4/1
  Constant1/1 -> Product1/1
  Gain/1 -> Add1/4
  u/1 -> Gain/1

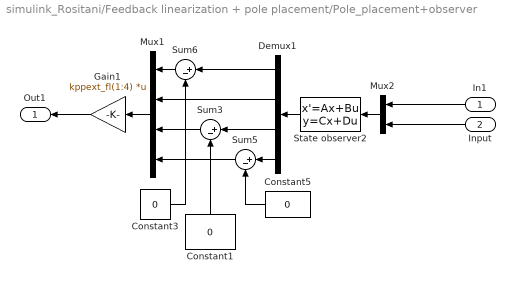
== system simulink_Rositani/Feedback linearization + pole placement/Pole_placement+observer ==
  In1 : Inport
  Input : Inport  Port=2
  Constant1 : Constant  Value=0
  Constant3 : Constant  Value=0
  Constant5 : Constant  Value=0
  Demux1 : Demux
  Gain1 : Gain  Gain=kppext_fl(1:4)  Multiplication=Matrix(K*u) (u vector)
  Mux1 : Mux
  Mux2 : Mux  Inputs=2
  State observer2 : StateSpace  A=M-Kobsfl*Cfl  B=[N-Kobsfl*Dfl Kobsfl]  C=eye(4)  D=[0 0;0 0;0 0;0 0]  InitialCondition=[pi/4 0 x3_bar 0]  ParameterTunability=Unconstrained
  Sum3 : Sum  Inputs=|+-
  Sum5 : Sum  Inputs=|+-
  Sum6 : Sum  Inputs=|+-
  Out1 : Outport
  wires:
  Constant3/1 -> Sum6/2
  Demux1/3 -> Sum3/1
  Mux2/1 -> State observer2/1
  In1/1 -> Mux2/1
  Constant5/1 -> Sum5/2
  State observer2/1 -> Demux1/1
  Demux1/2 -> Mux1/2
  Input/1 -> Mux2/2
  Sum3/1 -> Mux1/3
  Gain1/1 -> Out1/1
  Demux1/1 -> Sum6/1
  Mux1/1 -> Gain1/1
  Sum6/1 -> Mux1/1
  Demux1/4 -> Sum5/1
  Sum5/1 -> Mux1/4
  Constant1/1 -> Sum3/2

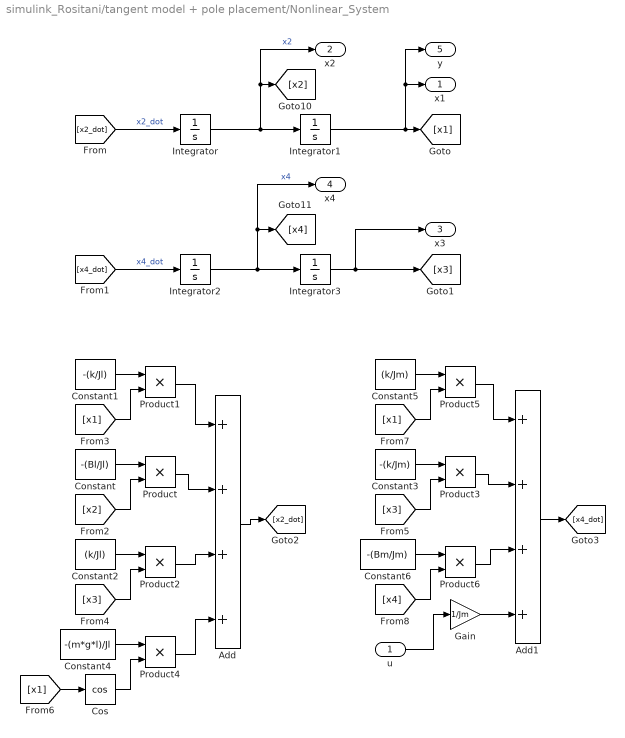
== system simulink_Rositani/tangent model + pole placement/Nonlinear_System ==
  u : Inport
  Add : Sum  Inputs=++++
  Add1 : Sum  Inputs=++++
  Constant : Constant  Value=-(Bl/Jl)
  Constant1 : Constant  Value=-(k/Jl)
  Constant2 : Constant  Value=(k/Jl)
  Constant3 : Constant  Value=-(k/Jm)
  Constant4 : Constant  Value=-(m*g*l)/Jl
  Constant5 : Constant  Value=(k/Jm)
  Constant6 : Constant  Value=-(Bm/Jm)
  Cos : Trigonometry  Operator=cos
  Gain : Gain  Gain=1/Jm
  Integrator : Integrator  InitialCondition=x0(2)
  Integrator1 : Integrator  InitialCondition=x0(1)
  Integrator2 : Integrator  InitialCondition=x0(4)
  Integrator3 : Integrator  InitialCondition=x0(3)
  Product{,1..6} (7 alike) : Product
  x1 : Outport
  x2 : Outport  Port=2
  x3 : Outport  Port=3
  x4 : Outport  Port=4
  y : Outport  Port=5
  wires:
  [x2] -> Product/2
  [x2_dot] -> Integrator/1  "x2_dot"
  [x1] -> Product1/2
  Constant2/1 -> Product2/1
  [x1] -> Product5/2
  Product1/1 -> Add/1
  [x4] -> Product6/2
  Product3/1 -> Add1/2
  Integrator3/1 -> x3/1, [x3]
  [x4_dot] -> Integrator2/1  "x4_dot"
  [x3] -> Product2/2
  Constant6/1 -> Product6/1
  Cos/1 -> Product4/2
  Integrator1/1 -> y/1, x1/1, [x1]
  Integrator2/1 -> x4/1, [x4], Integrator3/1  "x4"
  Constant/1 -> Product/1
  Integrator/1 -> x2/1, [x2], Integrator1/1  "x2"
  [x1] -> Cos/1
  Product5/1 -> Add1/1
  Constant3/1 -> Product3/1
  Constant5/1 -> Product5/1
  Product/1 -> Add/2
  Product6/1 -> Add1/3
  Product2/1 -> Add/3
  Add/1 -> [x2_dot]
  [x3] -> Product3/2
  Product4/1 -> Add/4
  Add1/1 -> [x4_dot]
  Constant4/1 -> Product4/1
  Constant1/1 -> Product1/1
  Gain/1 -> Add1/4
  u/1 -> Gain/1
